simulink model "stream_fft"  (R2023a)
settings: Solver=VariableStepAuto  StartTime=0.0  StopTime=0  RelTol=1e-3
model workspace (MAT data in the model file):
  FFT_len = 2048
undefined symbols (not defined in the file): None, S, vsva2197, xcvc1902
libraries: aieBasic x4, dspsrcs4 x2, aieUtilities x2, dspxfrm3 x1, aieDSP x1, vmcUtilities x1
settings Model: Creator=ravidapu  LastModifiedBy=robg
settings SolverCC: AlgebraicLoopSolver=TrustRegion
settings DebuggingCC: UnconnectedInputMsg=warning  UnconnectedOutputMsg=warning  UnconnectedLineMsg=warning
settings ModelReferenceCC: EnableRefExpFcnMdlSchedulingChecks=on
settings RTWCC: DLArmComputeVersion=19.05

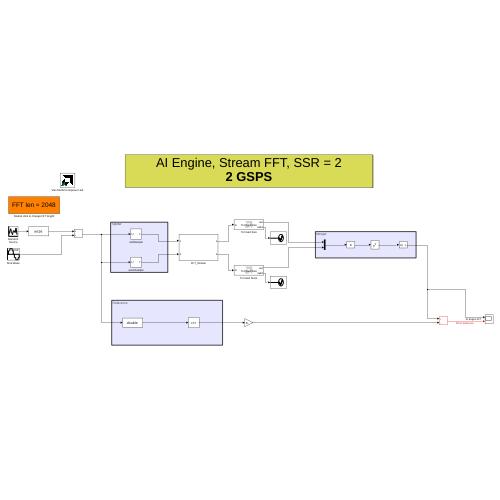
[thumbnail: Simulink's stored preview of the top-level diagram]
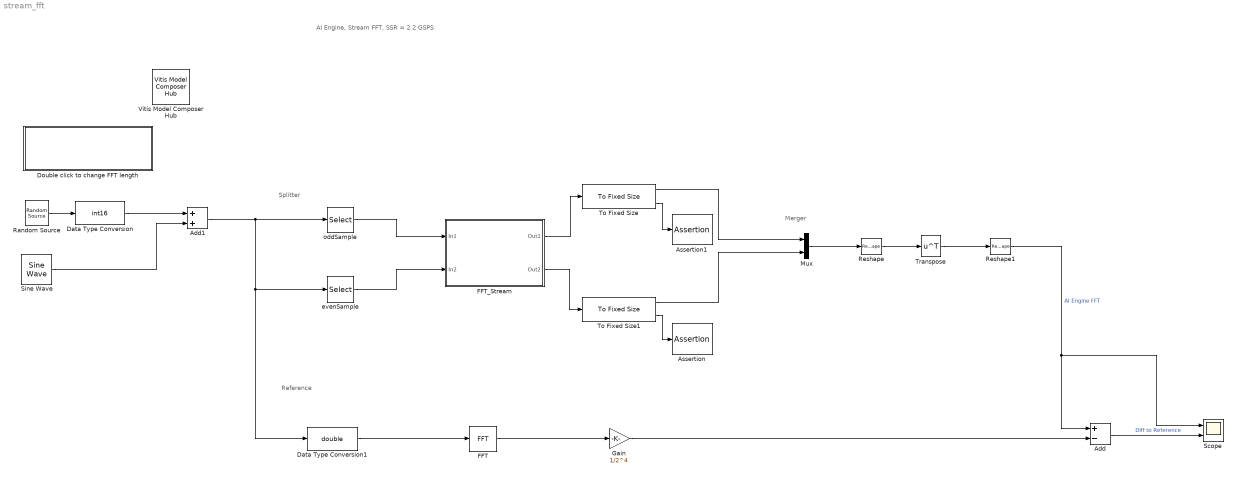
== system stream_fft ==
  note: Reference
  note: Splitter
  note: Merger
  note: AI Engine, Stream FFT, SSR = 2
      | 2 GSPS
  Add : Sum  Inputs=+-  OutDataTypeStr=double
  Add1 : Sum
  Assertion : Assertion
  Assertion1 : Assertion
  Data Type Conversion : DataTypeConversion  OutDataTypeStr=int16  SaturateOnIntegerOverflow=off  RndMeth=Floor
  Data Type Conversion1 : DataTypeConversion  OutDataTypeStr=double  SaturateOnIntegerOverflow=off  RndMeth=Floor
  Double click to change FFT length : Subsystem  mask{FFTlength=2048}
      mask prompts: FFTlength "FFT"
      mask help: Set the FFT length
      mask TypeOptions FFTlength: 128 | 256 | 512 | 1024 | 2048 | 4096
      mask Callback FFTlength:
      | FFTlen = str2double(get_param(gcb,'FFTlength'));
      | hws = get_param(bdroot, 'modelworkspace');
      | hws.assignin('FFT_len', FFTlen);
      mask Display:
      | FFTlen = get_param(gcb,'FFTlength');
      | disp(['\fontsize{24}FFT len = ' FFTlen ], 'texmode', 'on');
  FFT : dspxfrm3/FFT  FFTImplementation=Auto  CompMethod=Table lookup  TableOpt=NEW  TableOptActive=Speed  BitRevOrder=off  Normalize=off  InheritFFTLength=on  FFTLength=64  WrapInput=on  roundingMode=Floor  overflowMode=off  firstCoeffDataTypeStr=Inherit: Same word length as input  firstCoeffLastDataTypeStr=Inherit: Same word length as input  outputMin=[]  outputMax=[]
  FFT_Stream : Subsystem
  Gain : Gain  Gain=1/2^4
  Mux : Mux  Inputs=2
  Random Source : dspsrcs4/Random Source  SrcType=Uniform  NormMethod=Ziggurat  CltLength=12  MinVal=-5  MaxVal=5  MeanVal=0  VarVal=1  RepMode=Not repeatable  rawSeed=1  IsInherit=off  SampMode=Discrete  SampTime=1  SampFrame=FFT_len  DataType=Double  OutComplex=Complex  OutputFrames=off
  Reshape : Reshape  OutputDimensionality=Customize  OutputDimensions=[FFT_len/2, 2]
  Reshape1 : Reshape  OutputDimensions=[1, 10]
  Scope : Scope  NumInputPorts=2
  Sine Wave : dspsrcs4/Sine Wave  Amplitude=50  Frequency=1/10  Phase=0  SampleMode=Discrete  OutComplex=Real  CompMethod=Table lookup  TableSize=Speed  SampleTime=1  SamplesPerFrame=FFT_len  ResetState=Restart at time zero  OutputFrames=off  dataType=Fixed-point  wordLen=16  udDataType=sfix(16)  fracBitsMode=User-defined  numFracBits=0  OutDataTypeStr=fixdt(1,16,0)  LastOutDataTypeStr=fixdt(1,16,0)
  To Fixed Size : aieUtilities/To Fixed Size  Mode=Produce a valid output signal  OutputSize=Inherit: Same as input  CopyMethod=Buffer samples to form output  HasStatusOutput=off
  To Fixed Size1 : aieUtilities/To Fixed Size  Mode=Produce a valid output signal  OutputSize=Inherit: Same as input  CopyMethod=Buffer samples to form output  HasStatusOutput=off
  Transpose : Math  Operator=transpose
  Vitis Model Composer Hub : vmcUtilities/Vitis Model Composer Hub  Tag=genX  CodeGeneration=off  SubsystemName=FFT_Stream  StartColumn=1  NumberOfColumns=1  TargetDirectory=./code6  exportDesign=off  analyzeDesign=off  validateDesignOnHw=off  ExportType=AI Engines  IpVendor=xilinx.com  IpLibrary=hls  IpVersion=1.0  IpHWLanguage=Verilog  AieCompilerOptions={}  AieSimulatorOptions={}  CreateTestbench=on  TestbenchStackSize=10  RunRtlSim=off  RunCSim=off  RunAieSim=on  AieSimTimeout=50000  RunAieSimProfiling=off  LaunchVitisAnalyzer=on  PlotOutput=on  RunX86Sim=off  X86SimTimeout=10  GenHwImage=off  GenLibadfXo=off  GenHwValidationCode=off  PlatformType=Not Specified  HwSystemType=Baremetal  HwValidationTarget=hw  ProjDevice=xcvc1902-vsva2197-1LP-e-S  ProjDevicePart=xcvc1902-vsva2197-1LP-e-S  AIEType=AIE  SamplePeriod=-1  ClockFrequency=200  DataPathParallelism=1  xilinxfamily=Kintex7  part=xc7k325t  speed=-3  package=fbg676  directory=./netlist  testbench=off  incr_netlist=off  synthesis_tool=Vivado  clock_wrapper=Clock Enables  dbl_ovrd=According to Block Masks  dcm_input_clock_period=10  sysclk_period=10  simulink_period=1  eval_field=0  LogFileName=''  NThreads=4
  evenSample : Selector  InputPortWidth=FFT_len  IndexOptions=Index vector (dialog)  Indices=2:2:FFT_len  OutputSizes=1
  oddSample : Selector  InputPortWidth=FFT_len  IndexOptions=Index vector (dialog)  Indices=1:2:FFT_len  OutputSizes=1
  wires:
  evenSample/1 -> FFT_Stream/2(In2)
  FFT_Stream/1(Out1) -> To Fixed Size/1
  FFT_Stream/2(Out2) -> To Fixed Size1/1
  Reshape1/1 -> Add/1, Scope/1  "AI Engine FFT"
  FFT/1 -> Gain/1
  To Fixed Size/1 -> Mux/1
  Transpose/1 -> Reshape1/1
  Reshape/1 -> Transpose/1
  Mux/1 -> Reshape/1
  To Fixed Size1/1 -> Mux/2
  Add/1 -> Scope/2  "Diff to Reference"
  Data Type Conversion/1 -> Add1/1
  Add1/1 -> oddSample/1, evenSample/1, Data Type Conversion1/1
  Sine Wave/1 -> Add1/2
  Random Source/1 -> Data Type Conversion/1
  Data Type Conversion1/1 -> FFT/1
  To Fixed Size1/2 -> Assertion/1
  To Fixed Size/2 -> Assertion1/1
  Gain/1 -> Add/2
  oddSample/1 -> FFT_Stream/1(In1)

== system stream_fft/Double click to change FFT length ==

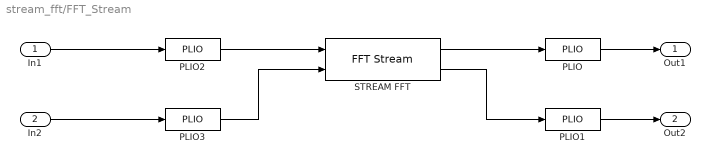
== system stream_fft/FFT_Stream ==
  In1 : Inport
  In2 : Inport  Port=2
  PLIO{,1..3} (4 alike) : aieBasic/PLIO  PlioWidth=64  PlioFreqSpec=on  PlioFreq=500  ColLocation=0  channel=0  blockJsonConstraints=[]  deprecateConstraints=0
  STREAM FFT : aieDSP/FFT Stream  AIE_VARIANT=1  data_type=cint16  data_out_type=cint16  twiddle_type=cint16  point_size=FFT_len  input_window_size=FFT_len  shift_val=4  rnd_mode=Round to positive infinity  sat_mode=0-None  ssr=2  twiddle_mode=0  use_ssr_widget_kernels=off  casc_length=1  blockJsonConstraints=[]  blockJsonConstraintsInternal=[]  spec=vmc_stream_fft.json  SerializedMaskParamNames=[]  SerializedMaskParamValues=[]  SerializedMaskParamVisibilities=[]  block_type=FFT Stream  SerializedMaskParamDataypes=uint|typename|typename|typename|uint|uint|uint|uint|uint|uint|uint|bool|uint  SerializedMaskParamEnumStrArr=0|0|0|0|0|0|0|Round to positive infinity,Round to negative infinity,Round symmetrical to infinity,Round symmetrical to zero,Round convergent to even,Round convergent to odd|0-None,1-Asymmetric,3-Symmetric|0|0|0|0  SerializedMaskParamEnumValArr=0|0|0|0|0|0|0|2,3,4,5,6,7|0,1,3|0|0|0|0  SerializedMaskParamVectorArr=0|0|0|0|0|0|0|0|0|0|0|0|0
  Out1 : Outport
  Out2 : Outport  Port=2
  wires:
  In1/1 -> PLIO2/1
  STREAM FFT/2 -> PLIO1/1
  STREAM FFT/1 -> PLIO/1
  In2/1 -> PLIO3/1
  PLIO/1 -> Out1/1
  PLIO1/1 -> Out2/1
  PLIO2/1 -> STREAM FFT/1
  PLIO3/1 -> STREAM FFT/2
